simulink model "ball"  (R2022a)
settings: Solver=VariableStepAuto  StartTime=0.0  StopTime=1  RelTol=1e-3
settings Model: Creator=User  LastModifiedBy=User

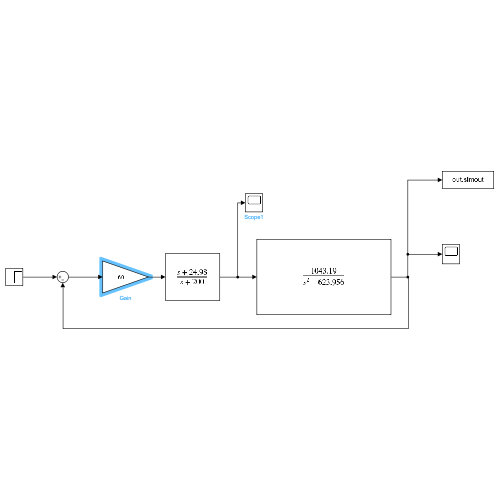
[thumbnail: Simulink's stored preview of the top-level diagram]
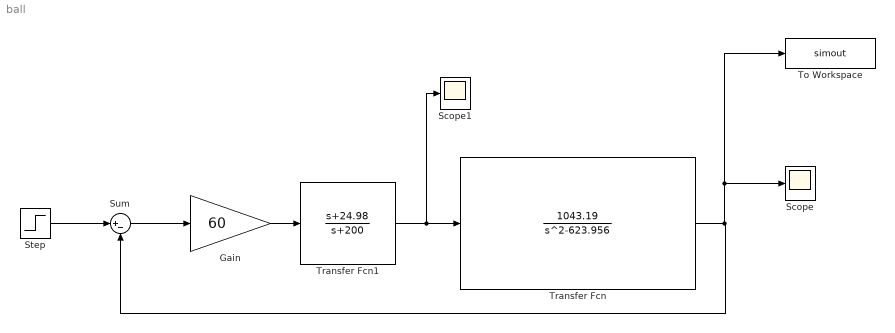
== system ball ==
  Gain : Gain  Gain=60
  Scope : Scope
  Scope1 : Scope
  Step : Step  Time=0  SampleTime=0
  Sum : Sum  Inputs=|+-
  To Workspace : ToWorkspace  VariableName=simout  SaveFormat=Timeseries  SampleTime=-1
      settings: Save2DSignal=2-D array (concatenate along first dimension)
  Transfer Fcn : TransferFcn  Numerator=[1043.19]  Denominator=[1 0 -623.956]
  Transfer Fcn1 : TransferFcn  Numerator=[1 24.98]  Denominator=[1 200]
  wires:
  Transfer Fcn/1 -> To Workspace/1, Scope/1, Sum/2
  Gain/1 -> Transfer Fcn1/1
  Step/1 -> Sum/1
  Sum/1 -> Gain/1
  Transfer Fcn1/1 -> Scope1/1, Transfer Fcn/1
